simulink model "semi6_2_indirect_diy"  (R2023a)
settings: Solver=VariableStepAuto  StartTime=0.0  StopTime=0.4  MaxStep=1e-3  RelTol=1e-3
libraries: spsIGBTDiodeLib x4, spsACVoltageSourceLib x1, spsDCVoltageSourceLib x1, spsFourierLib x1, spsCurrentMeasurementLib x1, spsRMSLib x1, spsSeriesRLCBranchLib x1, spsVoltageMeasurementLib x1, spspowerguiLib x1
settings Model: Creator=DELL  LastModifiedBy=11094
settings DataIOCC: ReturnWorkspaceOutputs=off
settings OptimizationCC: ReuseModelBlockBuffer=off
settings DebuggingCC: UnconnectedInputMsg=warning  UnconnectedOutputMsg=warning  UnconnectedLineMsg=warning
settings ModelReferenceCC: EnableRefExpFcnMdlSchedulingChecks=on
settings RTWCC: DLArmComputeVersion=19.05

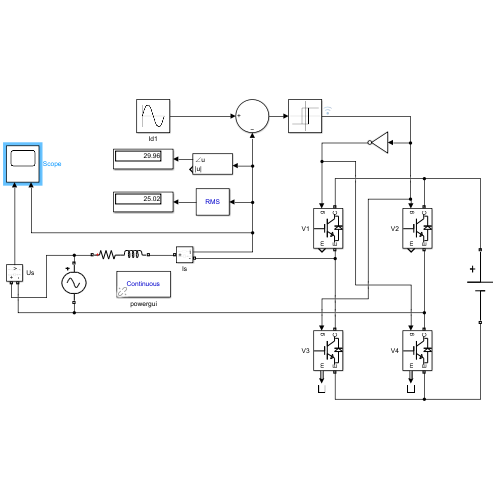
[thumbnail: Simulink's stored preview of the top-level diagram]
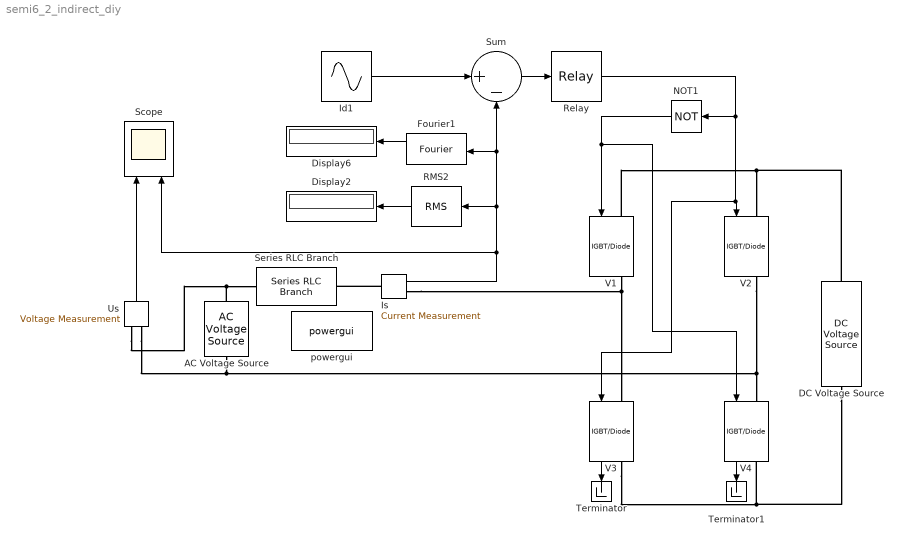
== system semi6_2_indirect_diy ==
  AC Voltage Source : spsACVoltageSourceLib/AC Voltage Source  Amplitude=220*sqrt(2)  Phase=0  Frequency=50  SampleTime=0  Measurements=None  BusType=swing  Pref=10e3  Qref=0  Qmin=-inf  Qmax=+inf
  DC Voltage Source : spsDCVoltageSourceLib/DC Voltage Source  Amplitude=550  Measurements=None
  Display2 : Display
  Display6 : Display
  Fourier1 : spsFourierLib/Fourier  Freq=50  n=1  InInit=[0, 0]  Ts=50e-8
  Id1 : Sin  Amplitude=25*sqrt(2)  Frequency=100*pi  Phase=30*pi/180  SampleTime=0
  Is : spsCurrentMeasurementLib/Current Measurement  PhasorSimulation=off  OutputType=Complex  PSBequivalent=0
  NOT1 : Logic  Operator=NOT  IconShape=distinctive  AllPortsSameDT=off  OutDataTypeStr=boolean
  RMS2 : spsRMSLib/RMS  TrueRMS=off  Freq=50  RMSInit=0  Ts=50e-8
  Relay : Relay  ZeroCross=off
  Scope : Scope  NumInputPorts=2
  Series RLC Branch : spsSeriesRLCBranchLib/Series RLC Branch  LConnTagsString=__new0  RConnTagsString=__new0  BranchType=RL  Resistance=0  Inductance=4e-3  SetiL0=off  InitialCurrent=0  Capacitance=1e-6  Setx0=off  InitialVoltage=0  Measurements=None
  Sum : Sum  Inputs=|+-
  Terminator : Terminator
  Terminator1 : Terminator
  Us : spsVoltageMeasurementLib/Voltage Measurement  PhasorSimulation=off  OutputType=Complex  PSBequivalent=0
  V{1..4} (4 alike) : spsIGBTDiodeLib/IGBT//Diode  Ron=1e-3  Rs=1e5  Cs=inf  Measurements=on
  powergui : spspowerguiLib/powergui  Priority=1  SimulationMode=Continuous  SampleTime=50e-8  frequency=60  Iterations=50  frequencyindice=50  Pbase=100e6  ErrMax=1e-4  UnitsV=kV  UnitsW=MW  buscounter=0  FunctionMessages=off  echomessages=off  EnableUseOfTLC=off  CurrentSourceSwitches=off  DisableSnubberDevices=off  DisableRonSwitches=off  DisableVfSwitches=off  DisplayEquations=off  AutomaticDiscreteSolvers=off  SolverType=Tustin/Backward Euler (TBE)  Interpol=off  ExternalGateDelay=off  methode=off  Ts=100  x0status=blocks  SPID=on  SwTol=0  HookPort=off  NonlinearTolerance=1e-4  nMaxIteration=100  ContinueOnMaxIteration=off  RestoreLinks=warning  ResistiveCurrentMeasurement=off  Frange=[0:2:500]  Ylog=off  Xlog=on  ShowGrid=off  save=off  variable=ZData  structure=0  ZoomFFT=off  StartTime=0.0  cycles=1  DisplayStyle=1  fundamental=60  FreqAxis=off  MaxFrequency=1000  frequencyindicesteady=1  RmsSteady=1  display=off
  wires:
  Fourier1/2 -> Display6/1
  V4/1 -> Terminator1/1
  RMS2/1 -> Display2/1
  V3/1 -> Terminator/1
  Is/1 -> Sum/2, Fourier1/1, RMS2/1, Scope/2
  Id1/1 -> Sum/1
  Sum/1 -> Relay/1
  Relay/1 -> NOT1/1, V2/1, V3/1
  NOT1/1 -> V4/1, V1/1
  Us/1 -> Scope/1
  connections:
  Is/LConn1 -- Series RLC Branch/RConn1
  AC Voltage Source/LConn1 -- Us/LConn2 -- V4/LConn1 -- V2/RConn1
  V3/RConn1 -- DC Voltage Source/LConn1 -- V4/RConn1
  V1/LConn1 -- DC Voltage Source/RConn1 -- V2/LConn1
  AC Voltage Source/RConn1 -- Us/LConn1 -- Series RLC Branch/LConn1
  Is/RConn1 -- V1/RConn1 -- V3/LConn1
